simulink model "simulink_estanques_sinxd"  (R2021a)
settings: Solver=ode1  StartTime=0.0  StopTime=500  FixedStep=0.001  RelTol=1e-3
settings Model: Creator=danie  LastModifiedBy=herr_df

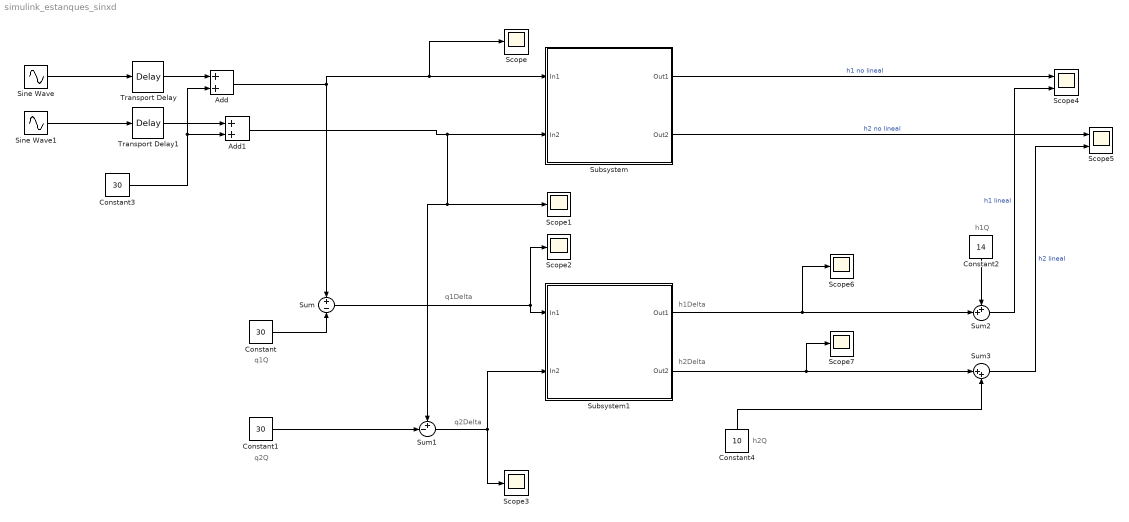
== system simulink_estanques_sinxd ==
  note: h2Delta
  note: h1Delta
  note: h1Q
  note: q1Delta
  note: q2Delta
  note: q2Q
  note: q1Q
  note: h2Q
  Add : Sum
  Add1 : Sum
  Constant : Constant  Value=30
  Constant1 : Constant  Value=30
  Constant2 : Constant  Value=14
  Constant3 : Constant  Value=30
  Constant4 : Constant  Value=10
  Scope{,1..3,6..7} (6 alike) : Scope
  Scope4 : Scope  NumInputPorts=2
  Scope5 : Scope  NumInputPorts=2
  Sine Wave : Sin  Amplitude=0  Bias=5  Frequency=0  SampleTime=0
  Sine Wave1 : Sin  Amplitude=0  Bias=15  Frequency=0  SampleTime=0
  Subsystem : Subsystem  mask{K=15, A=100, h10=14, h20=10}
      mask prompts: K "Coeficente de Traspaso"; A "Área Basal"; h10 "Altura inicial 1"; h20 "Altura inicial 2"
      mask Display:
      | port_label('input',1,'q1');
      | port_label('input',2,'q2');
      | port_label('output',1,'h1');
      | port_label('output',2,'h2');
      | fprintf('Sistema No lineal');
  Subsystem1 : Subsystem  mask{h2q=10, h1q=14, gamma=15/(2*(14-10)), K=15, A=100}
      mask prompts: K "Ka"; A "Área Basal"
      mask Display:
      | port_label('input',1,'q1');
      | port_label('input',2,'q2');
      | port_label('output',1,'h1');
      | port_label('output',2,'h2');
      | fprintf('Sistema Lineal');
  Sum : Sum  Inputs=+|-
  Sum1 : Sum  Inputs=+-|
  Sum2 : Sum  Inputs=++|
  Sum3 : Sum  Inputs=|++
  Transport Delay : TransportDelay  DelayTime=5
  Transport Delay1 : TransportDelay  DelayTime=5
  wires:
  Sine Wave/1 -> Transport Delay/1
  Sine Wave1/1 -> Transport Delay1/1
  Sum/1 -> Scope2/1, Subsystem1/1(In1)
  Constant/1 -> Sum/2
  Constant1/1 -> Sum1/2
  Sum1/1 -> Subsystem1/2(In2), Scope3/1
  Subsystem1/2(Out2) -> Sum3/1, Scope7/1
  Subsystem1/1(Out1) -> Scope6/1, Sum2/2
  Constant4/1 -> Sum3/2
  Constant2/1 -> Sum2/1
  Sum2/1 -> Scope4/2  "h1 lineal"
  Subsystem/1(Out1) -> Scope4/1  "h1 no lineal"
  Subsystem/2(Out2) -> Scope5/1  "h2 no lineal"
  Sum3/1 -> Scope5/2  "h2 lineal"
  Transport Delay/1 -> Add/1
  Add/1 -> Scope/1, Subsystem/1(In1), Sum/1
  Constant3/1 -> Add1/2, Add/2
  Transport Delay1/1 -> Add1/1
  Add1/1 -> Sum1/1, Scope1/1, Subsystem/2(In2)

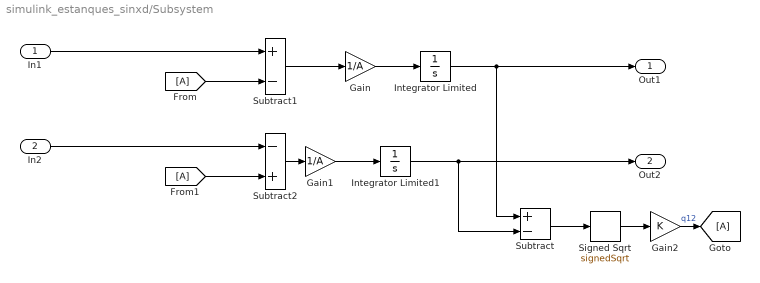
== system simulink_estanques_sinxd/Subsystem ==
  In1 : Inport
  In2 : Inport  Port=2
  Gain : Gain  Gain=1/A
  Gain1 : Gain  Gain=1/A
  Gain2 : Gain  Gain=K
  Integrator Limited : Integrator  InitialCondition=h10  LimitOutput=on  UpperSaturationLimit=500  LowerSaturationLimit=0
  Integrator Limited1 : Integrator  InitialCondition=h20  LimitOutput=on  UpperSaturationLimit=500  LowerSaturationLimit=0
  Signed Sqrt : Sqrt  Operator=signedSqrt  SaturateOnIntegerOverflow=on
  Subtract : Sum  Inputs=+-
  Subtract1 : Sum  Inputs=+-
  Subtract2 : Sum  Inputs=-+
  Out1 : Outport
  Out2 : Outport  Port=2
  wires:
  Subtract/1 -> Signed Sqrt/1
  Signed Sqrt/1 -> Gain2/1
  In1/1 -> Subtract1/1
  Gain2/1 -> [A]  "q12"
  [A] -> Subtract1/2
  [A] -> Subtract2/2
  In2/1 -> Subtract2/1
  Integrator Limited/1 -> Subtract/1, Out1/1
  Subtract1/1 -> Gain/1
  Gain/1 -> Integrator Limited/1
  Subtract2/1 -> Gain1/1
  Gain1/1 -> Integrator Limited1/1
  Integrator Limited1/1 -> Out2/1, Subtract/2

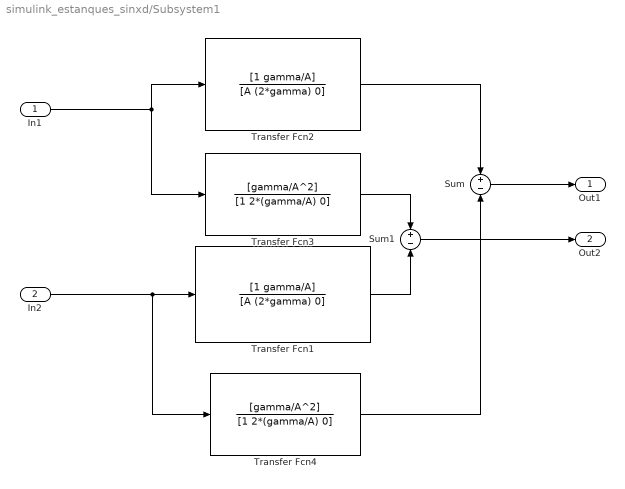
== system simulink_estanques_sinxd/Subsystem1 ==
  In1 : Inport
  In2 : Inport  Port=2
  Sum : Sum  Inputs=+|-
  Sum1 : Sum  Inputs=+|-
  Transfer Fcn1 : TransferFcn  Numerator=[1 gamma/A]  Denominator=[A (2*gamma) 0]
  Transfer Fcn2 : TransferFcn  Numerator=[1 gamma/A]  Denominator=[A (2*gamma) 0]
  Transfer Fcn3 : TransferFcn  Numerator=[gamma/A^2]  Denominator=[1 2*(gamma/A) 0]
  Transfer Fcn4 : TransferFcn  Numerator=[gamma/A^2]  Denominator=[1 2*(gamma/A) 0]
  Out1 : Outport
  Out2 : Outport  Port=2
  wires:
  In1/1 -> Transfer Fcn3/1, Transfer Fcn2/1
  Transfer Fcn2/1 -> Sum/1
  Transfer Fcn3/1 -> Sum1/1
  Sum/1 -> Out1/1
  Sum1/1 -> Out2/1
  In2/1 -> Transfer Fcn4/1, Transfer Fcn1/1
  Transfer Fcn1/1 -> Sum1/2
  Transfer Fcn4/1 -> Sum/2
